simulink model "OBC_MIL"  (R2024a)
settings: Solver=VariableStepAuto  StartTime=0.0  StopTime=inf  RelTol=1e-3
libraries: simulink x1
settings Model: Creator=crazy_racer  LastModifiedBy=ASUS
settings SolverCC: AlgebraicLoopSolver=TrustRegion
settings DebuggingCC: UnconnectedInputMsg=warning  UnconnectedOutputMsg=warning  UnconnectedLineMsg=warning
settings ModelReferenceCC: EnableRefExpFcnMdlSchedulingChecks=on
settings RTWCC: GPUComputeCapability=3.5

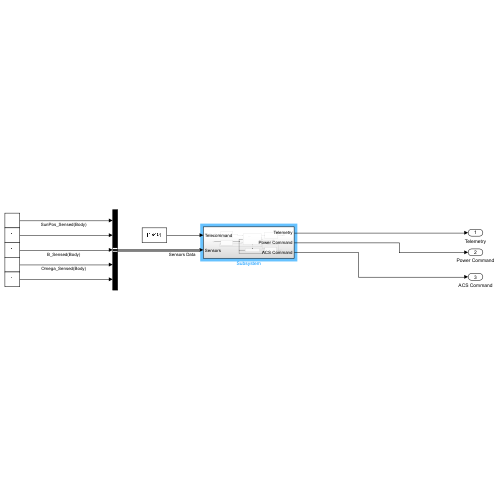
[thumbnail: Simulink's stored preview of the top-level diagram]
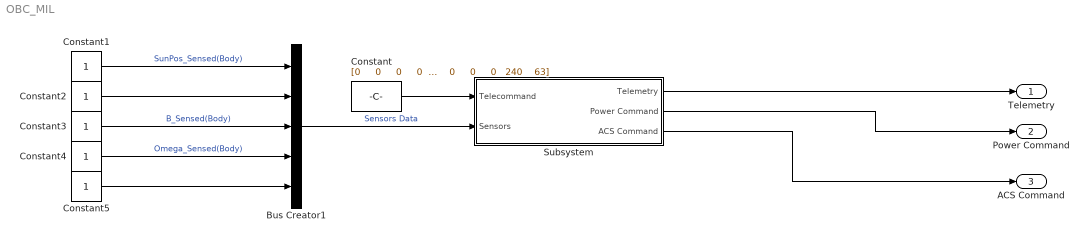
== system OBC_MIL ==
  Bus Creator1 : BusCreator  Inputs=5
  Constant : Constant  Value="[0     0     0     0     0     0   240    63     0     0     0     0     0     0     0     0     0     0     0     0 0     0     0     0     0     0     0     0     0     0     0     0     0     0     0     0     0     0   240    63]"  OutDataTypeStr=uint8
  Constant{1..5} (5 alike) : Constant
  Subsystem : Subsystem
  Telemetry : Outport
  Power Command : Outport  Port=2
  ACS Command : Outport  Port=3
  wires:
  Bus Creator1/1 -> Subsystem/2(Sensors)  "Sensors Data"
  Subsystem/1(Telemetry) -> Telemetry/1
  Subsystem/2(Power Command) -> Power Command/1
  Subsystem/3(ACS Command) -> ACS Command/1
  Constant/1 -> Subsystem/1(Telecommand)
  Constant3/1 -> Bus Creator1/3  "B_Sensed(Body)"
  Constant1/1 -> Bus Creator1/1  "SunPos_Sensed(Body)"
  Constant4/1 -> Bus Creator1/4  "Omega_Sensed(Body)"
  Constant5/1 -> Bus Creator1/5
  Constant2/1 -> Bus Creator1/2

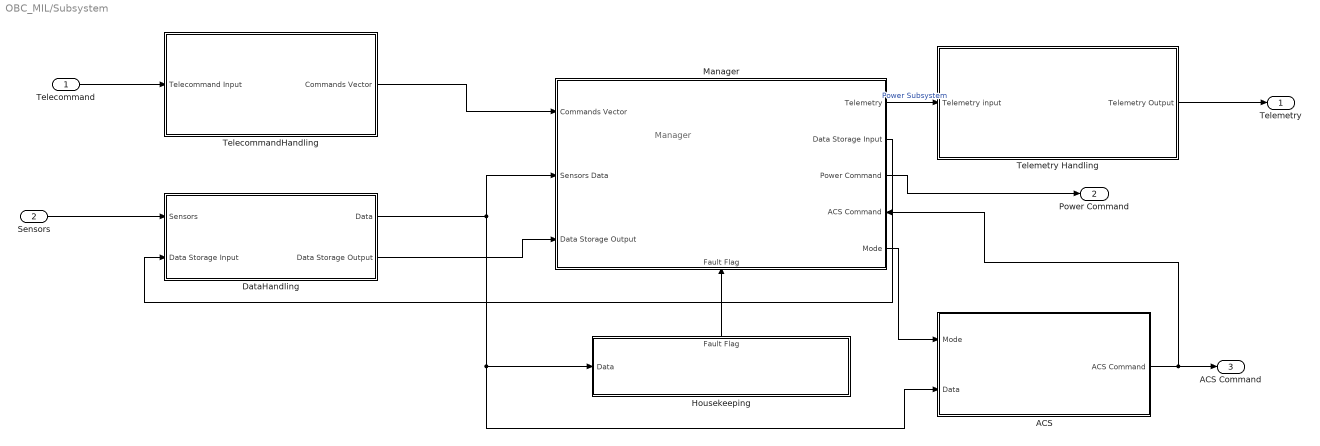
== system OBC_MIL/Subsystem ==
  note: Manager
  Telecommand : Inport
  Sensors : Inport  Port=2
  " Manager" : Subsystem
      settings: PortSchema="{\"entries\":[{\"content\":{\"sides\":[{\"content\":{\"connectorIds\":[\"In1\",\"In2\",\"In3\"]},\"type\":\"ConnectorPlacement.EquallySpacedRectSide\",\"uuid\":\"ec07d368-8191-42e4-9375-c2c602df22cf\"},{\"content\":{\"connectorIds\":[\"Out1\",\"Out2\",\"Out3\",\"In5\",\"Out4\"],\"side\":\"RIGHT\"},\"type\":\"ConnectorPlacement.EquallySpacedRectSide\",\"uuid\":\"bfabc2f5-2100-4bb6-919b-28e5c4a4cd4f\"},{\"content\":{\"side\":\"TOP\"},\"type\":\"ConnectorPlacement.EquallySpacedRectSide\",\"uuid\":\"1116e096-0190-44f1-9e3d-e2304f4178f6\"},{\"content\":{\"connectorIds\":[\"In4\"],\"side\":\"BOTTOM\"},\"type\":\"ConnectorPlacement.EquallySpacedRectSide\",\"uuid\":\"3d921d5d-5d93-4419-baa2-2f36ac6a4a99\"}]},\"type\":\"ConnectorPlacement.EquallySpacedConnector\",\"uuid\":\"03acd5cc-f7c7-46e5-a21e-c8fb7c082571\"}],\"packageUris\":[\"http://schema.mathworks.com/mf0/Connector/R2020b\"],\"version\":\"1.0\"}"
  ACS : Subsystem
  DataHandling : Subsystem
  Housekeeping : Subsystem
      settings: PortSchema="{\"entries\":[{\"content\":{\"sides\":[{\"content\":{\"connectorIds\":[\"In1\"]},\"type\":\"ConnectorPlacement.EquallySpacedRectSide\",\"uuid\":\"8eabc5dd-b460-4602-97d0-241e39b04916\"},{\"content\":{\"side\":\"RIGHT\"},\"type\":\"ConnectorPlacement.EquallySpacedRectSide\",\"uuid\":\"34fc1683-6b23-42e6-b522-0d805f5ee3a0\"},{\"content\":{\"connectorIds\":[\"Out1\"],\"side\":\"TOP\"},\"type\":\"ConnectorPlacement.EquallySpacedRectSide\",\"uuid\":\"2e5f843e-dd0f-45a3-97ce-c55e6bc4c9fd\"}]},\"type\":\"ConnectorPlacement.EquallySpacedConnector\",\"uuid\":\"4787b5c4-2ae8-477e-a21f-abe35d36bbd4\"}],\"packageUris\":[\"http://schema.mathworks.com/mf0/Connector/R2020b\"],\"version\":\"1.0\"}"
  TelecommandHandling : Subsystem
  Telemetry Handling : Subsystem
  Telemetry : Outport
  Power Command : Outport  Port=2
  ACS Command : Outport  Port=3
  wires:
  " Manager"/1(Telemetry) -> Telemetry Handling/1(Telemetry input)  "Power Subsystem"
  Telecommand/1 -> TelecommandHandling/1(Telecommand Input)
  DataHandling/1(Data) -> ACS/2(Data), Housekeeping/1("Data "), " Manager"/2(Sensors Data)
  TelecommandHandling/1(Commands Vector) -> " Manager"/1(Commands Vector)
  " Manager"/2(Data Storage Input) -> DataHandling/2(Data Storage Input)
  Housekeeping/1(Fault Flag) -> " Manager"/4(Fault Flag)
  " Manager"/3(Power Command) -> Power Command/1
  Telemetry Handling/1(Telemetry Output) -> Telemetry/1
  Sensors/1 -> DataHandling/1(Sensors)
  DataHandling/2(Data Storage Output) -> " Manager"/3(Data Storage Output)
  " Manager"/4(Mode) -> ACS/1(Mode)
  ACS/1(ACS Command) -> " Manager"/5(ACS Command), ACS Command/1

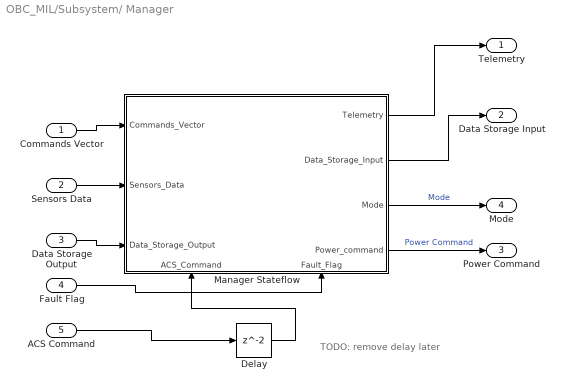
== system OBC_MIL/Subsystem/ Manager ==
  note: TODO: remove delay later
  Commands Vector : Inport
  Sensors Data : Inport  Port=2
  Data Storage Output : Inport  Port=3
  Fault Flag : Inport  Port=4
  ACS Command : Inport  Port=5
  Delay : Delay
  Manager Stateflow : Stateflow chart  TreatAsAtomicUnit=on
      settings: PortSchema="{\"entries\":[{\"content\":{\"sides\":[{\"content\":{\"connectorIds\":[\"In3\",\"In4\",\"In5\"]},\"type\":\"ConnectorPlacement.EquallySpacedRectSide\",\"uuid\":\"e1f10b30-4f11-427f-80a1-99253ceb8573\"},{\"content\":{\"connectorIds\":[\"Out1\",\"Out3\",\"Out4\",\"Out2\"],\"side\":\"RIGHT\"},\"type\":\"ConnectorPlacement.EquallySpacedRectSide\",\"uuid\":\"4c8c458e-9418-464f-accf-2ac8778338cd\"},{\"content\":{\"side\":\"TOP\"},\"type\":\"ConnectorPlacement.EquallySpacedRectSide\",\"uuid\":\"e00657ff-7d3d-45d1-9d17-1dfc8ef8ce11\"},{\"content\":{\"connectorIds\":[\"In1\",\"In2\"],\"side\":\"BOTTOM\"},\"type\":\"ConnectorPlacement.EquallySpacedRectSide\",\"uuid\":\"427faea7-f341-40f5-a655-462f7a6a3110\"}]},\"type\":\"ConnectorPlacement.EquallySpacedConnector\",\"uuid\":\"4ecfb0d2-db40-4a9e-b203-98a08a8aa01e\"}],\"packageUris\":[\"http://schema.mathworks.com/mf0/Connector/R2020b\"],\"version\":\"1.0\"}"
  Telemetry : Outport
  Data Storage Input : Outport  Port=2
  Power Command : Outport  Port=3
  Mode : Outport  Port=4
  wires:
  Commands Vector/1 -> Manager Stateflow/3(Commands_Vector)
  Sensors Data/1 -> Manager Stateflow/4(Sensors_Data)
  Data Storage Output/1 -> Manager Stateflow/5(Data_Storage_Output)
  Manager Stateflow/1(Telemetry) -> Telemetry/1
  Manager Stateflow/3(Data_Storage_Input) -> Data Storage Input/1
  Manager Stateflow/2(Power_command) -> Power Command/1  "Power Command"
  Fault Flag/1 -> Manager Stateflow/2(Fault_Flag)
  Manager Stateflow/4(Mode) -> Mode/1  "Mode"
  ACS Command/1 -> Delay/1
  Delay/1 -> Manager Stateflow/1(ACS_Command)

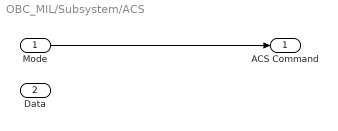
== system OBC_MIL/Subsystem/ACS ==
  Mode : Inport
  Data : Inport  Port=2
  ACS Command : Outport
  wires:
  Mode/1 -> ACS Command/1

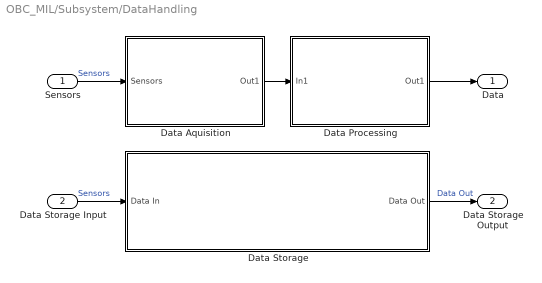
== system OBC_MIL/Subsystem/DataHandling ==
  Sensors : Inport
  Data Storage Input : Inport  Port=2
  Data Aquisition : Subsystem
  Data Processing : Subsystem
  Data Storage : Subsystem
  Data : Outport
  Data Storage Output : Outport  Port=2
  wires:
  Data Aquisition/1(Out1) -> Data Processing/1(In1)
  Sensors/1 -> Data Aquisition/1(Sensors)  "Sensors"
  Data Storage/1(Data Out) -> Data Storage Output/1  "Data Out"
  Data Processing/1(Out1) -> Data/1
  Data Storage Input/1 -> Data Storage/1(Data In)  "Sensors"

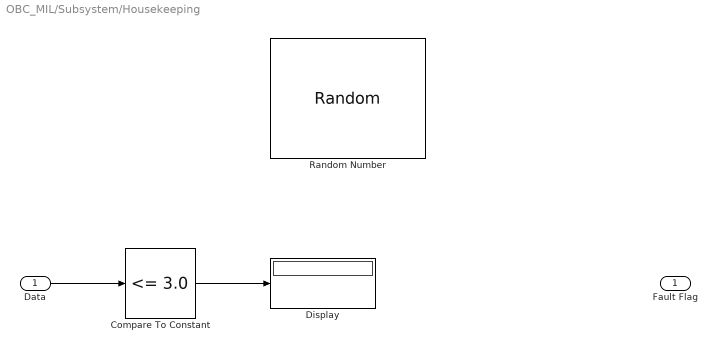
== system OBC_MIL/Subsystem/Housekeeping ==
  "Data " : Inport
  Compare To Constant : simulink/Logic and Bit Operations/Compare To Constant  relop=<=  const=3.0  OutDataTypeStr=boolean
  Display : Display
  Random Number : RandomNumber  SampleTime=100
  Fault Flag : Outport
  wires:
  "Data "/1 -> Compare To Constant/1
  Compare To Constant/1 -> Display/1

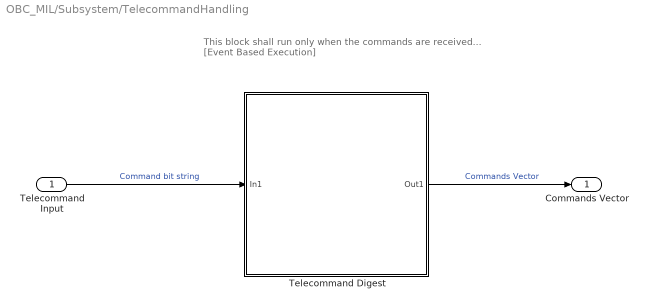
== system OBC_MIL/Subsystem/TelecommandHandling ==
  note: This block shall run only when the commands
      |  are received... [Event Based Execution]
  Telecommand Input : Inport
  Telecommand Digest : Subsystem
  Commands Vector : Outport
  wires:
  Telecommand Input/1 -> Telecommand Digest/1(In1)  "Command bit string"
  Telecommand Digest/1(Out1) -> Commands Vector/1  "Commands Vector"

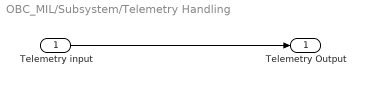
== system OBC_MIL/Subsystem/Telemetry Handling ==
  Telemetry input : Inport
  Telemetry Output : Outport
  wires:
  Telemetry input/1 -> Telemetry Output/1

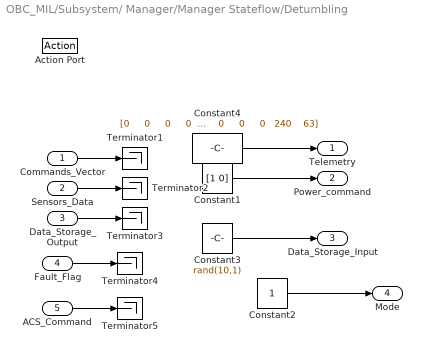
== system OBC_MIL/Subsystem/ Manager/Manager Stateflow/Detumbling ==
  Commands_Vector : Inport
  Sensors_Data : Inport  Port=2
  Data_Storage_Output : Inport  Port=3
  Fault_Flag : Inport  Port=4
  ACS_Command : Inport  Port=5
  Action Port : ActionPort
      settings: CopyFcn=Stateflow.SLINSF.SimulinkMan.removeBlockPreDeleteFcn  PreDeleteFcn=Stateflow.SLINSF.SimulinkMan.unsafePredeleteFcn
  Constant1 : Constant  Value=[1 0]  OutDataTypeStr=uint8
  Constant2 : Constant
  Constant3 : Constant  Value=rand(10,1)
  Constant4 : Constant  Value="[0     0     0     0     0     0   240    63     0     0     0     0     0     0     0     0     0     0     0     0 0     0     0     0     0     0     0     0     0     0     0     0     0     0     0     0     0     0   240    63]"  OutDataTypeStr=uint8
  Terminator{1..5} (5 alike) : Terminator
  Telemetry : Outport
  Power_command : Outport  Port=2
  Data_Storage_Input : Outport  Port=3
  Mode : Outport  Port=4
  wires:
  Commands_Vector/1 -> Terminator1/1
  Sensors_Data/1 -> Terminator2/1
  Data_Storage_Output/1 -> Terminator3/1
  Constant4/1 -> Telemetry/1
  Constant1/1 -> Power_command/1
  Constant3/1 -> Data_Storage_Input/1
  Fault_Flag/1 -> Terminator4/1
  ACS_Command/1 -> Terminator5/1
  Constant2/1 -> Mode/1

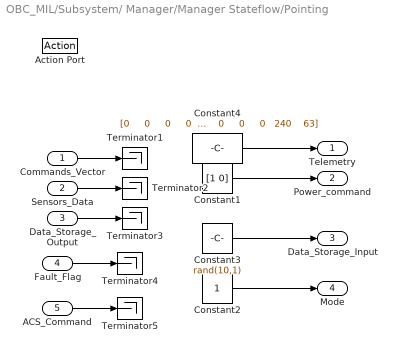
== system OBC_MIL/Subsystem/ Manager/Manager Stateflow/Pointing ==
  Commands_Vector : Inport
  Sensors_Data : Inport  Port=2
  Data_Storage_Output : Inport  Port=3
  Fault_Flag : Inport  Port=4
  ACS_Command : Inport  Port=5
  Action Port : ActionPort
      settings: CopyFcn=Stateflow.SLINSF.SimulinkMan.removeBlockPreDeleteFcn  PreDeleteFcn=Stateflow.SLINSF.SimulinkMan.unsafePredeleteFcn
  Constant1 : Constant  Value=[1 0]  OutDataTypeStr=uint8
  Constant2 : Constant
  Constant3 : Constant  Value=rand(10,1)
  Constant4 : Constant  Value="[0     0     0     0     0     0   240    63     0     0     0     0     0     0     0     0     0     0     0     0 0     0     0     0     0     0     0     0     0     0     0     0     0     0     0     0     0     0   240    63]"  OutDataTypeStr=uint8
  Terminator{1..5} (5 alike) : Terminator
  Telemetry : Outport
  Power_command : Outport  Port=2
  Data_Storage_Input : Outport  Port=3
  Mode : Outport  Port=4
  wires:
  Commands_Vector/1 -> Terminator1/1
  Sensors_Data/1 -> Terminator2/1
  Data_Storage_Output/1 -> Terminator3/1
  Constant4/1 -> Telemetry/1
  Constant1/1 -> Power_command/1
  Constant3/1 -> Data_Storage_Input/1
  Fault_Flag/1 -> Terminator4/1
  ACS_Command/1 -> Terminator5/1
  Constant2/1 -> Mode/1

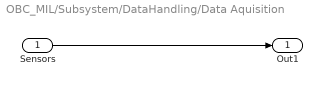
== system OBC_MIL/Subsystem/DataHandling/Data Aquisition ==
  Sensors : Inport
  Out1 : Outport
  wires:
  Sensors/1 -> Out1/1

== system OBC_MIL/Subsystem/DataHandling/Data Processing ==
  In1 : Inport
  Out1 : Outport
  wires:
  In1/1 -> Out1/1

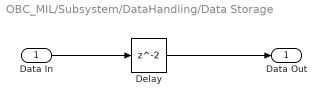
== system OBC_MIL/Subsystem/DataHandling/Data Storage ==
  Data In : Inport
  Delay : Delay
  Data Out : Outport
  wires:
  Data In/1 -> Delay/1
  Delay/1 -> Data Out/1

== system OBC_MIL/Subsystem/TelecommandHandling/Telecommand Digest ==
  In1 : Inport
  Out1 : Outport
  wires:
  In1/1 -> Out1/1

== stateflow chart OBC_MIL/Subsystem/ Manager/Manager Stateflow ==
  state Pointing
  state Detumbling
  state Boot
    mode_state = 2;
  Detumbling -> Pointing : [mode_state==2]
  Pointing -> Detumbling : [mode_state==1]
  Boot -> Detumbling : {mode_state = 2;}
  (default) -> Boot
  data: sf_internal_action_state_placeholder_data local double size=1 =0; sf_internal_action_state_placeholder_data local double size=1 =0; ACS_Command input; Fault_Flag input; Commands_Vector input; Sensors_Data input; Data_Storage_Output input; Telemetry output; Power_command output; Data_Storage_Input output; Mode output; mode_state local
